simulink model "counters"  (R2021a)
settings: Solver=VariableStepAuto  StartTime=0.0  StopTime=10.0  RelTol=1e-3
settings Model: Creator=NoteBook  LastModifiedBy=NoteBook

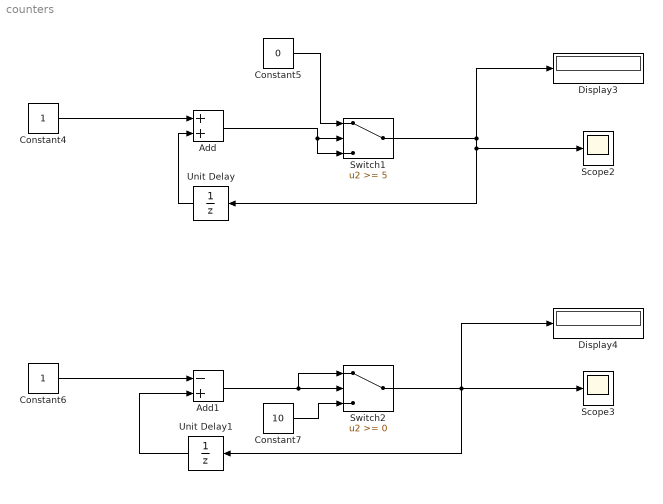
== system counters ==
  Add : Sum
  Add1 : Sum  Inputs=-+
  Constant4 : Constant  OutDataTypeStr=int16
  Constant5 : Constant  Value=0  OutDataTypeStr=int16
  Constant6 : Constant  OutDataTypeStr=int16
  Constant7 : Constant  Value=10  OutDataTypeStr=int16
  Display3 : Display
  Display4 : Display
  Scope2 : Scope
  Scope3 : Scope
  Switch1 : Switch  Threshold=5
  Switch2 : Switch
  Unit Delay : UnitDelay  SampleTime=-1  HasFrameUpgradeWarning=on
  Unit Delay1 : UnitDelay  SampleTime=-1  HasFrameUpgradeWarning=on
  wires:
  Constant7/1 -> Switch2/3
  Constant5/1 -> Switch1/1
  Add1/1 -> Switch2/1, Switch2/2
  Add/1 -> Switch1/3, Switch1/2
  Switch2/1 -> Scope3/1, Display4/1, Unit Delay1/1
  Constant6/1 -> Add1/1
  Unit Delay1/1 -> Add1/2
  Constant4/1 -> Add/1
  Unit Delay/1 -> Add/2
  Switch1/1 -> Unit Delay/1, Scope2/1, Display3/1
